simulink model "gm_ControllerTestbench"  (R2020b)
settings: Solver=VariableStepAuto  StartTime=0.0  StopTime=4  RelTol=1e-3
model workspace (MAT data in the model file):
  randSeedTorque = 0
  randomSeedSpeed = 0
undefined symbols (not defined in the file or in its folder): DiscIntNeverNeededParam, I_max, Position_PI_Limit
libraries: simulink x4, hdlmdlgenlib x1
(part 2 of 2)

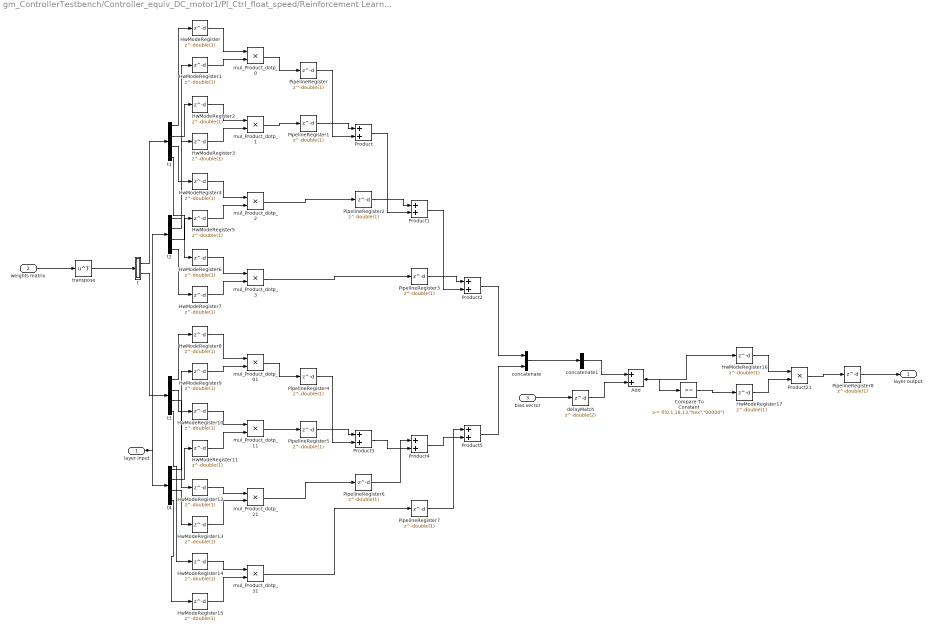
== system gm_ControllerTestbench/Controller_equiv_DC_motor1/PI_Ctrl_float_speed/Reinforcement Learning1/Subsystem Reference2/Hidden Layer (2 Neurons) ==
  layer input : Inport  OutDataTypeStr=fixdt(0, 18, 15)  PortDimensions=[4 1]  SampleTime=6.25e-05
  weights matrix : Inport  Port=2  OutDataTypeStr=fixdt(1, 18, 15)  PortDimensions=[2,4]  SampleTime=6.25e-05
  bias vector : Inport  Port=3  OutDataTypeStr=fixdt(0, 18, 18)  PortDimensions=[2 1]  SampleTime=6.25e-05
  Add : Sum  AccumDataTypeStr=fixdt(1, 32, 18)  OutDataTypeStr=fixdt(1, 18, 13)  SampleTime=6.25e-05
  Compare To Constant : simulink/Logic and Bit Operations/Compare To Constant  relop=>=  const="fi(0,1,18,13,\"hex\",\"00000\")"  OutDataTypeStr=boolean
  HwModeRegister{,1..17} (18 alike) : Delay  DelayLength=double(1)  InitialCondition=0  SampleTime=6.25e-05
  PipelineRegister{,1..8} (9 alike) : Delay  DelayLength=double(1)  InitialCondition=0  SampleTime=6.25e-05
  Product{,1..5} (6 alike) : Sum  AccumDataTypeStr=fixdt(1, 18, 13)  OutDataTypeStr=fixdt(1, 18, 13)  SampleTime=6.25e-05
  Product21 : Product  Inputs=**  OutDataTypeStr=fixdt(0, 18, 14)  SampleTime=6.25e-05
  concatenate : Concatenate
  concatenate1 : Concatenate  NumInputs=1  Mode=Multidimensional array  ConcatenateDimension=2
  delayMatch : Delay  DelayLength=double(2)  InitialCondition=0  SampleTime=6.25e-05
  mul_Product_dotp_{0..3,11,21,31} (7 alike) : Product  Inputs=**  OutDataTypeStr=fixdt(1, 18, 13)  SampleTime=6.25e-05
  mul_Product_dotp_01 : Product  Inputs=**  OutDataTypeStr=fixdt(1, 18, 13)  SampleTime=6.25e-05
  t : Subsystem
  t{1..4} (4 alike) : Demux
  transpose : Math  Operator=transpose  SaturateOnIntegerOverflow=on
  layer output : Outport
  wires:
  delayMatch/1 -> Add/2
  Add/1 -> Compare To Constant/1, HwModeRegister16/1
  Compare To Constant/1 -> HwModeRegister17/1
  concatenate1/1 -> Add/1
  PipelineRegister8/1 -> layer output/1
  transpose/1 -> t/1(in0)
  t/1(out0) -> t1/1
  t/2(out1) -> t3/1
  Product2/1 -> concatenate/1
  t1/1 -> HwModeRegister/1
  t1/2 -> HwModeRegister2/1
  t1/3 -> HwModeRegister4/1
  t1/4 -> HwModeRegister6/1
  t2/1 -> HwModeRegister1/1
  t2/2 -> HwModeRegister3/1
  t2/3 -> HwModeRegister5/1
  t2/4 -> HwModeRegister7/1
  PipelineRegister/1 -> Product/2
  PipelineRegister1/1 -> Product/1
  Product/1 -> Product1/2
  PipelineRegister2/1 -> Product1/1
  Product1/1 -> Product2/2
  PipelineRegister3/1 -> Product2/1
  Product5/1 -> concatenate/2
  t3/1 -> HwModeRegister8/1
  t3/2 -> HwModeRegister10/1
  t3/3 -> HwModeRegister12/1
  t3/4 -> HwModeRegister14/1
  t4/1 -> HwModeRegister9/1
  t4/2 -> HwModeRegister11/1
  t4/3 -> HwModeRegister13/1
  t4/4 -> HwModeRegister15/1
  PipelineRegister4/1 -> Product3/2
  PipelineRegister5/1 -> Product3/1
  Product3/1 -> Product4/2
  PipelineRegister6/1 -> Product4/1
  Product4/1 -> Product5/2
  PipelineRegister7/1 -> Product5/1
  concatenate/1 -> concatenate1/1
  layer input/1 -> t4/1, t2/1
  weights matrix/1 -> transpose/1
  bias vector/1 -> delayMatch/1
  mul_Product_dotp_0/1 -> PipelineRegister/1
  HwModeRegister/1 -> mul_Product_dotp_0/1
  HwModeRegister1/1 -> mul_Product_dotp_0/2
  mul_Product_dotp_1/1 -> PipelineRegister1/1
  HwModeRegister2/1 -> mul_Product_dotp_1/1
  HwModeRegister3/1 -> mul_Product_dotp_1/2
  mul_Product_dotp_2/1 -> PipelineRegister2/1
  HwModeRegister4/1 -> mul_Product_dotp_2/1
  HwModeRegister5/1 -> mul_Product_dotp_2/2
  mul_Product_dotp_3/1 -> PipelineRegister3/1
  HwModeRegister6/1 -> mul_Product_dotp_3/1
  HwModeRegister7/1 -> mul_Product_dotp_3/2
  mul_Product_dotp_01/1 -> PipelineRegister4/1
  HwModeRegister8/1 -> mul_Product_dotp_01/1
  HwModeRegister9/1 -> mul_Product_dotp_01/2
  mul_Product_dotp_11/1 -> PipelineRegister5/1
  HwModeRegister10/1 -> mul_Product_dotp_11/1
  HwModeRegister11/1 -> mul_Product_dotp_11/2
  mul_Product_dotp_21/1 -> PipelineRegister6/1
  HwModeRegister12/1 -> mul_Product_dotp_21/1
  HwModeRegister13/1 -> mul_Product_dotp_21/2
  mul_Product_dotp_31/1 -> PipelineRegister7/1
  HwModeRegister14/1 -> mul_Product_dotp_31/1
  HwModeRegister15/1 -> mul_Product_dotp_31/2
  Product21/1 -> PipelineRegister8/1
  HwModeRegister16/1 -> Product21/1
  HwModeRegister17/1 -> Product21/2

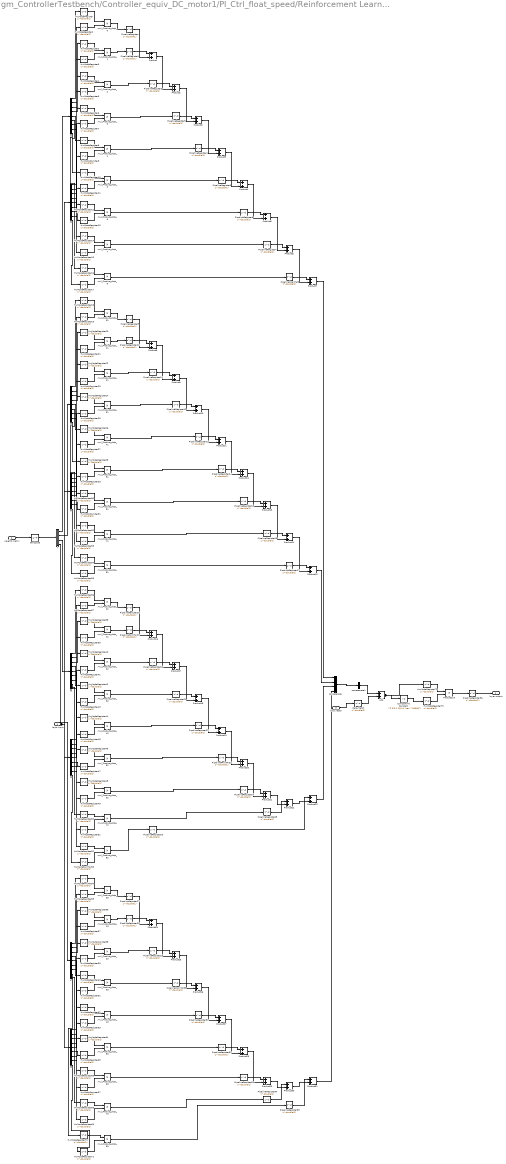
== system gm_ControllerTestbench/Controller_equiv_DC_motor1/PI_Ctrl_float_speed/Reinforcement Learning1/Subsystem Reference2/Input Layer (4 Neurons) ==
  layer input : Inport  OutDataTypeStr=fixdt(1, 18, 13)  PortDimensions=[9]  SampleTime=6.25e-05
  weights matrix : Inport  Port=2  OutDataTypeStr=fixdt(1, 18, 15)  PortDimensions=[4,9]  SampleTime=6.25e-05
  bias vector : Inport  Port=3  OutDataTypeStr=fixdt(1, 18, 17)  PortDimensions=[4 1]  SampleTime=6.25e-05
  Add : Sum  AccumDataTypeStr=fixdt(1, 32, 17)  OutDataTypeStr=fixdt(1, 18, 14)  SampleTime=6.25e-05
  Compare To Constant : simulink/Logic and Bit Operations/Compare To Constant  relop=>=  const="fi(0,1,18,14,\"hex\",\"00000\")"  OutDataTypeStr=boolean
  HwModeRegister{,1..73} (74 alike) : Delay  DelayLength=double(1)  InitialCondition=0  SampleTime=6.25e-05
  PipelineRegister{,1..36} (37 alike) : Delay  DelayLength=double(1)  InitialCondition=0  SampleTime=6.25e-05
  Product{,1..31} (32 alike) : Sum  AccumDataTypeStr=fixdt(1, 18, 14)  OutDataTypeStr=fixdt(1, 18, 14)  SampleTime=6.25e-05
  Product210 : Product  Inputs=**  OutDataTypeStr=fixdt(0, 18, 15)  SampleTime=6.25e-05
  concatenate : Concatenate  NumInputs=4
  concatenate1 : Concatenate  NumInputs=1  Mode=Multidimensional array  ConcatenateDimension=2
  delayMatch : Delay  DelayLength=double(2)  InitialCondition=0  SampleTime=6.25e-05
  mul_Product_dotp_{0..8,11..13,21..23,31..33,41..43,51..53,61..63,71..73,81..83} (33 alike) : Product  Inputs=**  OutDataTypeStr=fixdt(1, 18, 14)  SampleTime=6.25e-05
  mul_Product_dotp_01 : Product  Inputs=**  OutDataTypeStr=fixdt(1, 18, 14)  SampleTime=6.25e-05
  mul_Product_dotp_02 : Product  Inputs=**  OutDataTypeStr=fixdt(1, 18, 14)  SampleTime=6.25e-05
  mul_Product_dotp_03 : Product  Inputs=**  OutDataTypeStr=fixdt(1, 18, 14)  SampleTime=6.25e-05
  t : Subsystem
  t{1..8} (8 alike) : Demux  Outputs=9
  transpose : Math  Operator=transpose  SaturateOnIntegerOverflow=on
  layer output : Outport
  wires:
  delayMatch/1 -> Add/2
  Add/1 -> Compare To Constant/1, HwModeRegister72/1
  Compare To Constant/1 -> HwModeRegister73/1
  concatenate1/1 -> Add/1
  PipelineRegister36/1 -> layer output/1
  transpose/1 -> t/1(in0)
  t/1(out0) -> t1/1
  t/2(out1) -> t3/1
  t/3(out2) -> t5/1
  t/4(out3) -> t7/1
  Product7/1 -> concatenate/1
  t1/1 -> HwModeRegister/1
  t1/2 -> HwModeRegister2/1
  t1/3 -> HwModeRegister4/1
  t1/4 -> HwModeRegister6/1
  t1/5 -> HwModeRegister8/1
  t1/6 -> HwModeRegister10/1
  t1/7 -> HwModeRegister12/1
  t1/8 -> HwModeRegister14/1
  t1/9 -> HwModeRegister16/1
  t2/1 -> HwModeRegister1/1
  t2/2 -> HwModeRegister3/1
  t2/3 -> HwModeRegister5/1
  t2/4 -> HwModeRegister7/1
  t2/5 -> HwModeRegister9/1
  t2/6 -> HwModeRegister11/1
  t2/7 -> HwModeRegister13/1
  t2/8 -> HwModeRegister15/1
  t2/9 -> HwModeRegister17/1
  PipelineRegister/1 -> Product/2
  PipelineRegister1/1 -> Product/1
  Product/1 -> Product1/2
  PipelineRegister2/1 -> Product1/1
  Product1/1 -> Product2/2
  PipelineRegister3/1 -> Product2/1
  Product2/1 -> Product3/2
  PipelineRegister4/1 -> Product3/1
  Product3/1 -> Product4/2
  PipelineRegister5/1 -> Product4/1
  Product4/1 -> Product5/2
  PipelineRegister6/1 -> Product5/1
  Product5/1 -> Product6/2
  PipelineRegister7/1 -> Product6/1
  Product6/1 -> Product7/2
  PipelineRegister8/1 -> Product7/1
  Product15/1 -> concatenate/2
  t3/1 -> HwModeRegister18/1
  t3/2 -> HwModeRegister20/1
  t3/3 -> HwModeRegister22/1
  t3/4 -> HwModeRegister24/1
  t3/5 -> HwModeRegister26/1
  t3/6 -> HwModeRegister28/1
  t3/7 -> HwModeRegister30/1
  t3/8 -> HwModeRegister32/1
  t3/9 -> HwModeRegister34/1
  t4/1 -> HwModeRegister19/1
  t4/2 -> HwModeRegister21/1
  t4/3 -> HwModeRegister23/1
  t4/4 -> HwModeRegister25/1
  t4/5 -> HwModeRegister27/1
  t4/6 -> HwModeRegister29/1
  t4/7 -> HwModeRegister31/1
  t4/8 -> HwModeRegister33/1
  t4/9 -> HwModeRegister35/1
  PipelineRegister9/1 -> Product8/2
  PipelineRegister10/1 -> Product8/1
  Product8/1 -> Product9/2
  PipelineRegister11/1 -> Product9/1
  Product9/1 -> Product10/2
  PipelineRegister12/1 -> Product10/1
  Product10/1 -> Product11/2
  PipelineRegister13/1 -> Product11/1
  Product11/1 -> Product12/2
  PipelineRegister14/1 -> Product12/1
  Product12/1 -> Product13/2
  PipelineRegister15/1 -> Product13/1
  Product13/1 -> Product14/2
  PipelineRegister16/1 -> Product14/1
  Product14/1 -> Product15/2
  PipelineRegister17/1 -> Product15/1
  Product23/1 -> concatenate/3
  t5/1 -> HwModeRegister36/1
  t5/2 -> HwModeRegister38/1
  t5/3 -> HwModeRegister40/1
  t5/4 -> HwModeRegister42/1
  t5/5 -> HwModeRegister44/1
  t5/6 -> HwModeRegister46/1
  t5/7 -> HwModeRegister48/1
  t5/8 -> HwModeRegister50/1
  t5/9 -> HwModeRegister52/1
  t6/1 -> HwModeRegister37/1
  t6/2 -> HwModeRegister39/1
  t6/3 -> HwModeRegister41/1
  t6/4 -> HwModeRegister43/1
  t6/5 -> HwModeRegister45/1
  t6/6 -> HwModeRegister47/1
  t6/7 -> HwModeRegister49/1
  t6/8 -> HwModeRegister51/1
  t6/9 -> HwModeRegister53/1
  PipelineRegister18/1 -> Product16/2
  PipelineRegister19/1 -> Product16/1
  Product16/1 -> Product17/2
  PipelineRegister20/1 -> Product17/1
  Product17/1 -> Product18/2
  PipelineRegister21/1 -> Product18/1
  Product18/1 -> Product19/2
  PipelineRegister22/1 -> Product19/1
  Product19/1 -> Product20/2
  PipelineRegister23/1 -> Product20/1
  Product20/1 -> Product21/2
  PipelineRegister24/1 -> Product21/1
  Product21/1 -> Product22/2
  PipelineRegister25/1 -> Product22/1
  Product22/1 -> Product23/2
  PipelineRegister26/1 -> Product23/1
  Product31/1 -> concatenate/4
  t7/1 -> HwModeRegister54/1
  t7/2 -> HwModeRegister56/1
  t7/3 -> HwModeRegister58/1
  t7/4 -> HwModeRegister60/1
  t7/5 -> HwModeRegister62/1
  t7/6 -> HwModeRegister64/1
  t7/7 -> HwModeRegister66/1
  t7/8 -> HwModeRegister68/1
  t7/9 -> HwModeRegister70/1
  t8/1 -> HwModeRegister55/1
  t8/2 -> HwModeRegister57/1
  t8/3 -> HwModeRegister59/1
  t8/4 -> HwModeRegister61/1
  t8/5 -> HwModeRegister63/1
  t8/6 -> HwModeRegister65/1
  t8/7 -> HwModeRegister67/1
  t8/8 -> HwModeRegister69/1
  t8/9 -> HwModeRegister71/1
  PipelineRegister27/1 -> Product24/2
  PipelineRegister28/1 -> Product24/1
  Product24/1 -> Product25/2
  PipelineRegister29/1 -> Product25/1
  Product25/1 -> Product26/2
  PipelineRegister30/1 -> Product26/1
  Product26/1 -> Product27/2
  PipelineRegister31/1 -> Product27/1
  Product27/1 -> Product28/2
  PipelineRegister32/1 -> Product28/1
  Product28/1 -> Product29/2
  PipelineRegister33/1 -> Product29/1
  Product29/1 -> Product30/2
  PipelineRegister34/1 -> Product30/1
  Product30/1 -> Product31/2
  PipelineRegister35/1 -> Product31/1
  concatenate/1 -> concatenate1/1
  layer input/1 -> t8/1, t6/1, t4/1, t2/1
  weights matrix/1 -> transpose/1
  bias vector/1 -> delayMatch/1
  mul_Product_dotp_0/1 -> PipelineRegister/1
  HwModeRegister/1 -> mul_Product_dotp_0/1
  HwModeRegister1/1 -> mul_Product_dotp_0/2
  mul_Product_dotp_1/1 -> PipelineRegister1/1
  HwModeRegister2/1 -> mul_Product_dotp_1/1
  HwModeRegister3/1 -> mul_Product_dotp_1/2
  mul_Product_dotp_2/1 -> PipelineRegister2/1
  HwModeRegister4/1 -> mul_Product_dotp_2/1
  HwModeRegister5/1 -> mul_Product_dotp_2/2
  mul_Product_dotp_3/1 -> PipelineRegister3/1
  HwModeRegister6/1 -> mul_Product_dotp_3/1
  HwModeRegister7/1 -> mul_Product_dotp_3/2
  mul_Product_dotp_4/1 -> PipelineRegister4/1
  HwModeRegister8/1 -> mul_Product_dotp_4/1
  HwModeRegister9/1 -> mul_Product_dotp_4/2
  mul_Product_dotp_5/1 -> PipelineRegister5/1
  HwModeRegister10/1 -> mul_Product_dotp_5/1
  HwModeRegister11/1 -> mul_Product_dotp_5/2
  mul_Product_dotp_6/1 -> PipelineRegister6/1
  HwModeRegister12/1 -> mul_Product_dotp_6/1
  HwModeRegister13/1 -> mul_Product_dotp_6/2
  mul_Product_dotp_7/1 -> PipelineRegister7/1
  HwModeRegister14/1 -> mul_Product_dotp_7/1
  HwModeRegister15/1 -> mul_Product_dotp_7/2
  mul_Product_dotp_8/1 -> PipelineRegister8/1
  HwModeRegister16/1 -> mul_Product_dotp_8/1
  HwModeRegister17/1 -> mul_Product_dotp_8/2
  mul_Product_dotp_01/1 -> PipelineRegister9/1
  HwModeRegister18/1 -> mul_Product_dotp_01/1
  HwModeRegister19/1 -> mul_Product_dotp_01/2
  mul_Product_dotp_11/1 -> PipelineRegister10/1
  HwModeRegister20/1 -> mul_Product_dotp_11/1
  HwModeRegister21/1 -> mul_Product_dotp_11/2
  mul_Product_dotp_21/1 -> PipelineRegister11/1
  HwModeRegister22/1 -> mul_Product_dotp_21/1
  HwModeRegister23/1 -> mul_Product_dotp_21/2
  mul_Product_dotp_31/1 -> PipelineRegister12/1
  HwModeRegister24/1 -> mul_Product_dotp_31/1
  HwModeRegister25/1 -> mul_Product_dotp_31/2
  mul_Product_dotp_41/1 -> PipelineRegister13/1
  HwModeRegister26/1 -> mul_Product_dotp_41/1
  HwModeRegister27/1 -> mul_Product_dotp_41/2
  mul_Product_dotp_51/1 -> PipelineRegister14/1
  HwModeRegister28/1 -> mul_Product_dotp_51/1
  HwModeRegister29/1 -> mul_Product_dotp_51/2
  mul_Product_dotp_61/1 -> PipelineRegister15/1
  HwModeRegister30/1 -> mul_Product_dotp_61/1
  HwModeRegister31/1 -> mul_Product_dotp_61/2
  mul_Product_dotp_71/1 -> PipelineRegister16/1
  HwModeRegister32/1 -> mul_Product_dotp_71/1
  HwModeRegister33/1 -> mul_Product_dotp_71/2
  mul_Product_dotp_81/1 -> PipelineRegister17/1
  HwModeRegister34/1 -> mul_Product_dotp_81/1
  HwModeRegister35/1 -> mul_Product_dotp_81/2
  mul_Product_dotp_02/1 -> PipelineRegister18/1
  HwModeRegister36/1 -> mul_Product_dotp_02/1
  HwModeRegister37/1 -> mul_Product_dotp_02/2
  mul_Product_dotp_12/1 -> PipelineRegister19/1
  HwModeRegister38/1 -> mul_Product_dotp_12/1
  HwModeRegister39/1 -> mul_Product_dotp_12/2
  mul_Product_dotp_22/1 -> PipelineRegister20/1
  HwModeRegister40/1 -> mul_Product_dotp_22/1
  HwModeRegister41/1 -> mul_Product_dotp_22/2
  mul_Product_dotp_32/1 -> PipelineRegister21/1
  HwModeRegister42/1 -> mul_Product_dotp_32/1
  HwModeRegister43/1 -> mul_Product_dotp_32/2
  mul_Product_dotp_42/1 -> PipelineRegister22/1
  HwModeRegister44/1 -> mul_Product_dotp_42/1
  HwModeRegister45/1 -> mul_Product_dotp_42/2
  mul_Product_dotp_52/1 -> PipelineRegister23/1
  HwModeRegister46/1 -> mul_Product_dotp_52/1
  HwModeRegister47/1 -> mul_Product_dotp_52/2
  mul_Product_dotp_62/1 -> PipelineRegister24/1
  HwModeRegister48/1 -> mul_Product_dotp_62/1
  HwModeRegister49/1 -> mul_Product_dotp_62/2
  mul_Product_dotp_72/1 -> PipelineRegister25/1
  HwModeRegister50/1 -> mul_Product_dotp_72/1
  HwModeRegister51/1 -> mul_Product_dotp_72/2
  mul_Product_dotp_82/1 -> PipelineRegister26/1
  HwModeRegister52/1 -> mul_Product_dotp_82/1
  HwModeRegister53/1 -> mul_Product_dotp_82/2
  mul_Product_dotp_03/1 -> PipelineRegister27/1
  HwModeRegister54/1 -> mul_Product_dotp_03/1
  HwModeRegister55/1 -> mul_Product_dotp_03/2
  mul_Product_dotp_13/1 -> PipelineRegister28/1
  HwModeRegister56/1 -> mul_Product_dotp_13/1
  HwModeRegister57/1 -> mul_Product_dotp_13/2
  mul_Product_dotp_23/1 -> PipelineRegister29/1
  HwModeRegister58/1 -> mul_Product_dotp_23/1
  HwModeRegister59/1 -> mul_Product_dotp_23/2
  mul_Product_dotp_33/1 -> PipelineRegister30/1
  HwModeRegister60/1 -> mul_Product_dotp_33/1
  HwModeRegister61/1 -> mul_Product_dotp_33/2
  mul_Product_dotp_43/1 -> PipelineRegister31/1
  HwModeRegister62/1 -> mul_Product_dotp_43/1
  HwModeRegister63/1 -> mul_Product_dotp_43/2
  mul_Product_dotp_53/1 -> PipelineRegister32/1
  HwModeRegister64/1 -> mul_Product_dotp_53/1
  HwModeRegister65/1 -> mul_Product_dotp_53/2
  mul_Product_dotp_63/1 -> PipelineRegister33/1
  HwModeRegister66/1 -> mul_Product_dotp_63/1
  HwModeRegister67/1 -> mul_Product_dotp_63/2
  mul_Product_dotp_73/1 -> PipelineRegister34/1
  HwModeRegister68/1 -> mul_Product_dotp_73/1
  HwModeRegister69/1 -> mul_Product_dotp_73/2
  mul_Product_dotp_83/1 -> PipelineRegister35/1
  HwModeRegister70/1 -> mul_Product_dotp_83/1
  HwModeRegister71/1 -> mul_Product_dotp_83/2
  Product210/1 -> PipelineRegister36/1
  HwModeRegister72/1 -> Product210/1
  HwModeRegister73/1 -> Product210/2

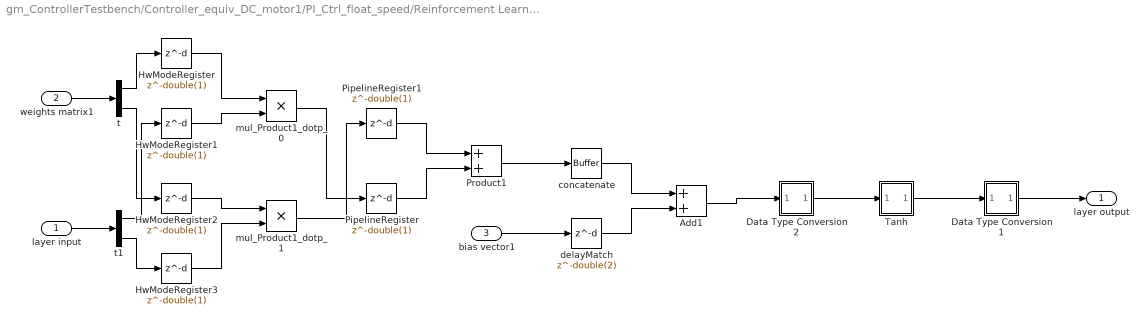
== system gm_ControllerTestbench/Controller_equiv_DC_motor1/PI_Ctrl_float_speed/Reinforcement Learning1/Subsystem Reference2/Output Layer (1 Neuron) ==
  layer input : Inport  OutDataTypeStr=fixdt(0, 18, 14)  PortDimensions=[2 1]  SampleTime=6.25e-05
  weights matrix1 : Inport  Port=2  OutDataTypeStr=fixdt(1, 18, 15)  PortDimensions=[1 2]  SampleTime=6.25e-05
  bias vector1 : Inport  Port=3  OutDataTypeStr=fixdt(0, 18, 18)  PortDimensions=1  SampleTime=6.25e-05
  Add1 : Sum  AccumDataTypeStr=fixdt(1, 18, 11)  OutDataTypeStr=fixdt(1, 18, 11)  SampleTime=6.25e-05
  Data Type Conversion1 : Subsystem
      mask Display: disp('NFP\nconv');
  Data Type Conversion2 : Subsystem
      mask Display: disp('NFP\nconv');
  HwModeRegister{,1..3} (4 alike) : Delay  DelayLength=double(1)  InitialCondition=0  SampleTime=6.25e-05
  PipelineRegister : Delay  DelayLength=double(1)  InitialCondition=0  SampleTime=6.25e-05
  PipelineRegister1 : Delay  DelayLength=double(1)  InitialCondition=0  SampleTime=6.25e-05
  Product1 : Sum  AccumDataTypeStr=fixdt(1, 18, 11)  OutDataTypeStr=fixdt(1, 18, 11)  SampleTime=6.25e-05
  Tanh : Subsystem
      mask Display: disp('NFP\ntrig');
  concatenate : hdlmdlgenlib/Buffer
      settings: SourceProductBaseCode=SL
  delayMatch : Delay  DelayLength=double(2)  InitialCondition=0  SampleTime=6.25e-05
  mul_Product1_dotp_0 : Product  Inputs=**  OutDataTypeStr=fixdt(1, 18, 11)  SampleTime=6.25e-05
  mul_Product1_dotp_1 : Product  Inputs=**  OutDataTypeStr=fixdt(1, 18, 11)  SampleTime=6.25e-05
  t : Demux  Outputs=2
  t1 : Demux  Outputs=2
  layer output : Outport
  wires:
  delayMatch/1 -> Add1/2
  Add1/1 -> Data Type Conversion2/1(In1)
  concatenate/1 -> Add1/1
  Product1/1 -> concatenate/1
  t/1 -> HwModeRegister/1
  t/2 -> HwModeRegister2/1
  t1/1 -> HwModeRegister1/1
  t1/2 -> HwModeRegister3/1
  PipelineRegister/1 -> Product1/2
  PipelineRegister1/1 -> Product1/1
  Data Type Conversion1/1(Out1) -> layer output/1
  Data Type Conversion2/1(Out1) -> Tanh/1(In1)
  Tanh/1(Out1) -> Data Type Conversion1/1(In1)
  layer input/1 -> t1/1
  weights matrix1/1 -> t/1
  bias vector1/1 -> delayMatch/1
  mul_Product1_dotp_0/1 -> PipelineRegister/1
  HwModeRegister/1 -> mul_Product1_dotp_0/1
  HwModeRegister1/1 -> mul_Product1_dotp_0/2
  mul_Product1_dotp_1/1 -> PipelineRegister1/1
  HwModeRegister2/1 -> mul_Product1_dotp_1/1
  HwModeRegister3/1 -> mul_Product1_dotp_1/2

== system gm_ControllerTestbench/Controller_equiv_DC_motor1/PI_Ctrl_float_speed/Reinforcement Learning1/Reward/integrate/limit_abs_value_of_integrator ==
  input : Inport
  abs_max : Inport  Port=2
  CmpLT : RelationalOperator  Operator=<  OutDataTypeStr=boolean  RndMeth=Nearest
  CmpLT1 : RelationalOperator  OutDataTypeStr=boolean  RndMeth=Nearest
  Switch : Switch  Criteria=u2 ~= 0  Threshold=Position_PI_Limit  ZeroCross=off
  Switch1 : Switch  Criteria=u2 ~= 0  Threshold=I_max  ZeroCross=off
  Unary Minus : UnaryMinus
  output : Outport
  wires:
  CmpLT1/1 -> Switch/2
  abs_max/1 -> Switch/1, CmpLT1/2, Unary Minus/1
  input/1 -> CmpLT1/1, Switch/3, CmpLT/1
  CmpLT/1 -> Switch1/2
  Switch/1 -> Switch1/3
  Switch1/1 -> output/1
  Unary Minus/1 -> Switch1/1, CmpLT/2

== system gm_ControllerTestbench/Controller_equiv_DC_motor1/PI_Ctrl_float_speed/Reinforcement Learning1/Subsystem Reference2/Hidden Layer (2 Neurons)/t ==
  in0 : Inport
  ColVec1 : Selector  NumberOfDimensions=2  IndexOptions=Select all,Index vector (dialog)  Indices=1,1  OutputSizes=1,1
  ColVec2 : Selector  NumberOfDimensions=2  IndexOptions=Select all,Index vector (dialog)  Indices=1,2  OutputSizes=1,1
  out0 : Outport
  out1 : Outport  Port=2
  wires:
  in0/1 -> ColVec1/1, ColVec2/1
  ColVec1/1 -> out0/1
  ColVec2/1 -> out1/1

== system gm_ControllerTestbench/Controller_equiv_DC_motor1/PI_Ctrl_float_speed/Reinforcement Learning1/Subsystem Reference2/Input Layer (4 Neurons)/t ==
  in0 : Inport
  ColVec1 : Selector  NumberOfDimensions=2  IndexOptions=Select all,Index vector (dialog)  Indices=1,1  OutputSizes=1,1
  ColVec2 : Selector  NumberOfDimensions=2  IndexOptions=Select all,Index vector (dialog)  Indices=1,2  OutputSizes=1,1
  ColVec3 : Selector  NumberOfDimensions=2  IndexOptions=Select all,Index vector (dialog)  Indices=1,3  OutputSizes=1,1
  ColVec4 : Selector  NumberOfDimensions=2  IndexOptions=Select all,Index vector (dialog)  Indices=1,4  OutputSizes=1,1
  out0 : Outport
  out1 : Outport  Port=2
  out2 : Outport  Port=3
  out3 : Outport  Port=4
  wires:
  in0/1 -> ColVec1/1, ColVec2/1, ColVec3/1, ColVec4/1
  ColVec1/1 -> out0/1
  ColVec2/1 -> out1/1
  ColVec3/1 -> out2/1
  ColVec4/1 -> out3/1

== system gm_ControllerTestbench/Controller_equiv_DC_motor1/PI_Ctrl_float_speed/Reinforcement Learning1/Subsystem Reference2/Output Layer (1 Neuron)/Data Type Conversion1 ==
  In1 : Inport
  Data Type Conversion1 : DataTypeConversion  OutDataTypeStr=fixdt(1, 18, 16)  RndMeth=Nearest  SampleTime=6.25e-05
  Data Type Conversion1_pd1 : Delay  DelayLength=6
  Out1 : Outport
  wires:
  In1/1 -> Data Type Conversion1/1
  Data Type Conversion1/1 -> Data Type Conversion1_pd1/1
  Data Type Conversion1_pd1/1 -> Out1/1

== system gm_ControllerTestbench/Controller_equiv_DC_motor1/PI_Ctrl_float_speed/Reinforcement Learning1/Subsystem Reference2/Output Layer (1 Neuron)/Data Type Conversion2 ==
  In1 : Inport
  Data Type Conversion2 : DataTypeConversion  OutDataTypeStr=single  RndMeth=Nearest  SampleTime=6.25e-05
  Data Type Conversion2_pd1 : Delay  DelayLength=6
  Out1 : Outport
  wires:
  In1/1 -> Data Type Conversion2/1
  Data Type Conversion2/1 -> Data Type Conversion2_pd1/1
  Data Type Conversion2_pd1/1 -> Out1/1

== system gm_ControllerTestbench/Controller_equiv_DC_motor1/PI_Ctrl_float_speed/Reinforcement Learning1/Subsystem Reference2/Output Layer (1 Neuron)/Tanh ==
  In1 : Inport
  Tanh : Trigonometry  Operator=tanh  SampleTime=6.25e-05
  Tanh_pd1 : Delay  DelayLength=43
  Out1 : Outport
  wires:
  In1/1 -> Tanh/1
  Tanh/1 -> Tanh_pd1/1
  Tanh_pd1/1 -> Out1/1
